simulink model "Examen2019"  (R2022b)
settings: Solver=VariableStepAuto  StartTime=0.0  StopTime=100  MaxStep=0.01  RelTol=1e-3
undefined symbols (not defined in the file): Kp, Td, Ti, Tt
settings Model: Creator=OMEN  LastModifiedBy=Pablo
settings RTWCC: GPUComputeCapability=5.0

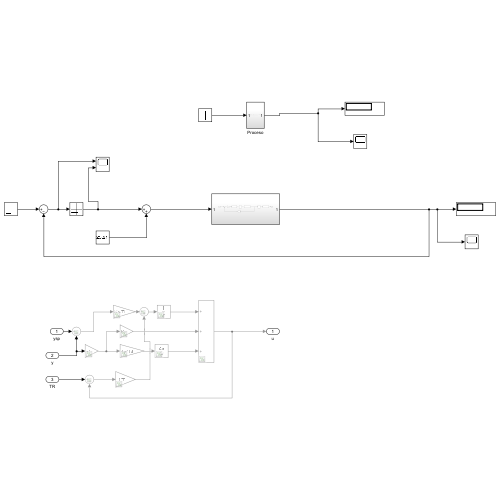
[thumbnail: Simulink's stored preview of the top-level diagram]
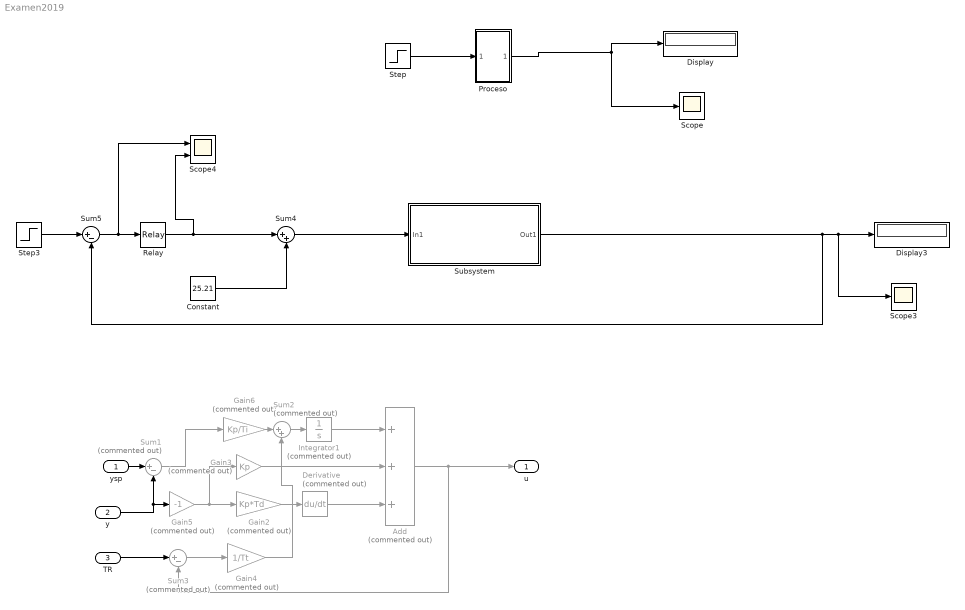
== system Examen2019 ==
  ysp : Inport
  y : Inport  Port=2
  TR : Inport  Port=3
  Add : Sum  Commented=on  Inputs=+++
  Constant : Constant  Value=25.21
  Derivative : Derivative  Commented=on
  Display : Display
  Display3 : Display
  Gain2 : Gain  Commented=on  Gain=Kp*Td
  Gain3 : Gain  Commented=on  Gain=Kp
  Gain4 : Gain  Commented=on  Gain=1/Tt
  Gain5 : Gain  Commented=on  Gain=-1
  Gain6 : Gain  Commented=on  Gain=Kp/Ti
  Integrator1 : Integrator  Commented=on
  Proceso : Subsystem
  Relay : Relay  OnOutputValue=5  OffOutputValue=-5
  Scope : Scope
  Scope3 : Scope
  Scope4 : Scope  NumInputPorts=2
  Step : Step  After=25.21  SampleTime=0
  Step3 : Step  After=160  SampleTime=0
  Subsystem : Subsystem
  Sum1 : Sum  Commented=on  Inputs=|+-
  Sum2 : Sum  Commented=on  Inputs=|++
  Sum3 : Sum  Commented=on  Inputs=|+-
  Sum4 : Sum  Inputs=|++
  Sum5 : Sum  Inputs=|+-
  u : Outport
  wires:
  Sum5/1 -> Scope4/1, Relay/1
  Step3/1 -> Sum5/1
  Subsystem/1(Out1) -> Sum5/2, Display3/1, Scope3/1
  Derivative/1 -> Add/3
  ysp/1 -> Sum1/1
  Add/1 -> Sum3/2, u/1
  Sum1/1 -> Gain6/1
  Gain2/1 -> Derivative/1
  Gain5/1 -> Gain3/1, Gain2/1
  y/1 -> Gain5/1, Sum1/2
  Integrator1/1 -> Add/1
  Gain3/1 -> Add/2
  Gain6/1 -> Sum2/1
  Sum2/1 -> Integrator1/1
  Gain4/1 -> Sum2/2
  TR/1 -> Sum3/1
  Sum3/1 -> Gain4/1
  Relay/1 -> Scope4/2, Sum4/1
  Sum4/1 -> Subsystem/1(In1)
  Constant/1 -> Sum4/2
  Proceso/1(Out1) -> Display/1, Scope/1
  Step/1 -> Proceso/1(In1)

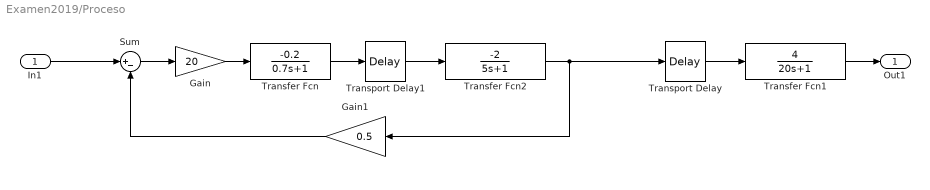
== system Examen2019/Proceso ==
  In1 : Inport
  Gain : Gain  Gain=20
  Gain1 : Gain  Gain=0.5
  Sum : Sum  Inputs=|+-
  Transfer Fcn : TransferFcn  Numerator=[-0.2]  Denominator=[0.7 1]
  Transfer Fcn1 : TransferFcn  Numerator=[4]  Denominator=[20 1]
  Transfer Fcn2 : TransferFcn  Numerator=[-2]  Denominator=[5 1]
  Transport Delay : TransportDelay  DelayTime=2
  Transport Delay1 : TransportDelay
  Out1 : Outport
  wires:
  Sum/1 -> Gain/1
  Transfer Fcn2/1 -> Gain1/1, Transport Delay/1
  Transport Delay1/1 -> Transfer Fcn2/1
  Transport Delay/1 -> Transfer Fcn1/1
  Transfer Fcn1/1 -> Out1/1
  Gain/1 -> Transfer Fcn/1
  Transfer Fcn/1 -> Transport Delay1/1
  Gain1/1 -> Sum/2
  In1/1 -> Sum/1

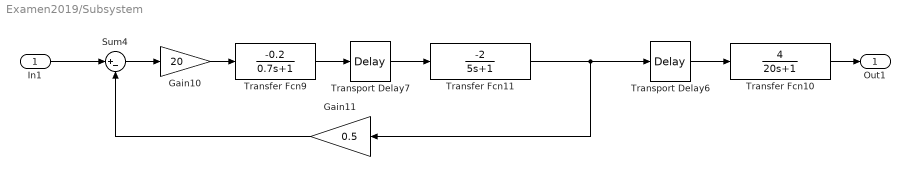
== system Examen2019/Subsystem ==
  In1 : Inport
  Gain10 : Gain  Gain=20
  Gain11 : Gain  Gain=0.5
  Sum4 : Sum  Inputs=|+-
  Transfer Fcn10 : TransferFcn  Numerator=[4]  Denominator=[20 1]
  Transfer Fcn11 : TransferFcn  Numerator=[-2]  Denominator=[5 1]
  Transfer Fcn9 : TransferFcn  Numerator=[-0.2]  Denominator=[0.7 1]
  Transport Delay6 : TransportDelay  DelayTime=2
  Transport Delay7 : TransportDelay
  Out1 : Outport
  wires:
  Transfer Fcn11/1 -> Gain11/1, Transport Delay6/1
  Transfer Fcn9/1 -> Transport Delay7/1
  Transport Delay6/1 -> Transfer Fcn10/1
  Gain11/1 -> Sum4/2
  Transport Delay7/1 -> Transfer Fcn11/1
  Sum4/1 -> Gain10/1
  Transfer Fcn10/1 -> Out1/1
  Gain10/1 -> Transfer Fcn9/1
  In1/1 -> Sum4/1
